simulink model "Fig-6-7-8"  (R2020b)
settings: Solver=VariableStepAuto  StartTime=0.0  StopTime=10.0  RelTol=1e-3
undefined symbols (not defined in the file or in its folder): drv, ms22g, sens, Ts
settings Model: Creator=piera  LastModifiedBy=piera

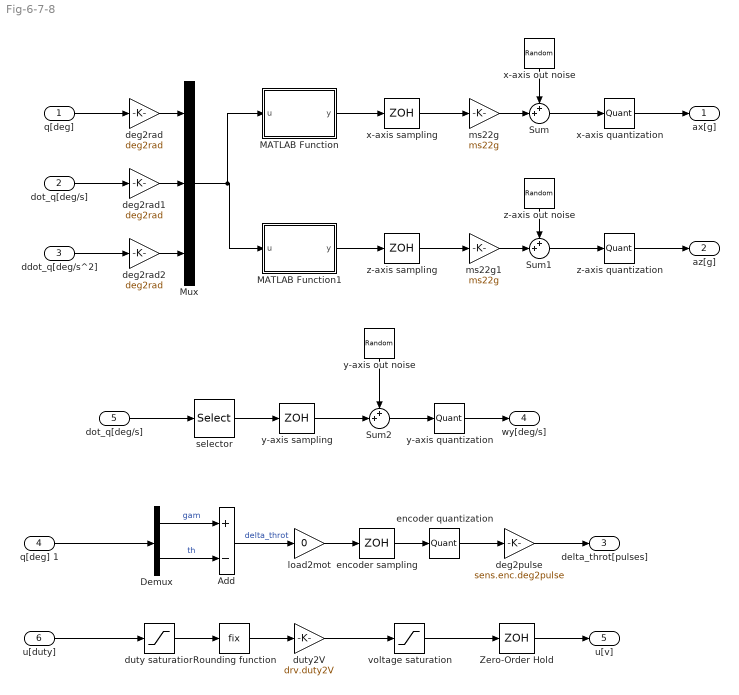
== system Fig-6-7-8 ==
  "q[deg] " : Inport
  dot_q[deg/s] : Inport  Port=2
  ddot_q[deg/s^2] : Inport  Port=3
  q[deg] 1 : Inport  Port=4
  "dot_q[deg/s] " : Inport  Port=5
  u[duty] : Inport  Port=6
  Add : Sum  Inputs=+-
  Demux : Demux  Outputs=2
  MATLAB Function : MATLAB Function  TreatAsAtomicUnit=on
  MATLAB Function1 : MATLAB Function  TreatAsAtomicUnit=on
  Mux : Mux  Inputs=3
  Rounding function : Rounding  Operator=fix
  Sum : Sum  Inputs=++|
  Sum1 : Sum  Inputs=++|
  Sum2 : Sum  Inputs=++|
  Zero-Order Hold : ZeroOrderHold  SampleTime=Ts
  deg2pulse : Gain  Gain=sens.enc.deg2pulse
  deg2rad : Gain  Gain=deg2rad
  deg2rad1 : Gain  Gain=deg2rad
  deg2rad2 : Gain  Gain=deg2rad
  duty saturation : Saturate  UpperLimit=drv.dutymax  LowerLimit=-drv.dutymax
  duty2V : Gain  Gain=drv.duty2V
  encoder quantization : Quantizer  QuantizationInterval=sens.enc.pulse2deg
  encoder sampling : ZeroOrderHold  SampleTime=Ts
  load2mot : Gain  Gain=0
  ms22g : Gain  Gain=ms22g
  ms22g1 : Gain  Gain=ms22g
  selector : Selector  InputPortWidth=2  IndexOptions=Index vector (dialog)  Indices=[2]  OutputSizes=1
  voltage saturation : Saturate  UpperLimit=drv.Vbus  LowerLimit=-drv.Vbus
  x-axis out noise : RandomNumber  Variance=sens.mpu.acc.noisevar  SampleTime=0.1
  x-axis quantization : Quantizer  QuantizationInterval=sens.mpu.acc.LSB2g
  x-axis sampling : ZeroOrderHold  SampleTime=-1
  y-axis out noise : RandomNumber  Variance=sens.mpu.gyro.noisevar  SampleTime=0.1
  y-axis quantization : Quantizer  QuantizationInterval=sens.mpu.gyro.LSB2g
  y-axis sampling : ZeroOrderHold  SampleTime=-1
  z-axis out noise : RandomNumber  Variance=sens.mpu.acc.noisevar  SampleTime=0.1
  z-axis quantization : Quantizer  QuantizationInterval=sens.mpu.acc.LSB2g
  z-axis sampling : ZeroOrderHold  SampleTime=-1
  ax[g] : Outport
  az[g] : Outport  Port=2
  delta_throt[pulses] : Outport  Port=3
  wy[deg/s] : Outport  Port=4
  u[v] : Outport  Port=5
  wires:
  deg2rad1/1 -> Mux/2
  deg2rad/1 -> Mux/1
  deg2rad2/1 -> Mux/3
  "q[deg] "/1 -> deg2rad/1
  dot_q[deg/s]/1 -> deg2rad1/1
  ddot_q[deg/s^2]/1 -> deg2rad2/1
  Mux/1 -> MATLAB Function/1(u), MATLAB Function1/1(u)
  MATLAB Function1/1(y) -> z-axis sampling/1
  MATLAB Function/1(y) -> x-axis sampling/1
  z-axis sampling/1 -> ms22g1/1
  x-axis sampling/1 -> ms22g/1
  ms22g/1 -> Sum/2
  x-axis out noise/1 -> Sum/1
  Sum/1 -> x-axis quantization/1
  x-axis quantization/1 -> ax[g]/1
  z-axis quantization/1 -> az[g]/1
  z-axis out noise/1 -> Sum1/1
  ms22g1/1 -> Sum1/2
  Sum1/1 -> z-axis quantization/1
  deg2pulse/1 -> delta_throt[pulses]/1
  encoder quantization/1 -> deg2pulse/1
  encoder sampling/1 -> encoder quantization/1
  load2mot/1 -> encoder sampling/1
  Add/1 -> load2mot/1  "delta_throt"
  q[deg] 1/1 -> Demux/1
  Demux/1 -> Add/1  "gam"
  Demux/2 -> Add/2  "th"
  y-axis quantization/1 -> wy[deg/s]/1
  Sum2/1 -> y-axis quantization/1
  y-axis out noise/1 -> Sum2/1
  y-axis sampling/1 -> Sum2/2
  selector/1 -> y-axis sampling/1
  "dot_q[deg/s] "/1 -> selector/1
  Zero-Order Hold/1 -> u[v]/1
  voltage saturation/1 -> Zero-Order Hold/1
  duty2V/1 -> voltage saturation/1
  Rounding function/1 -> duty2V/1
  duty saturation/1 -> Rounding function/1
  u[duty]/1 -> duty saturation/1

== matlab function Fig-6-7-8/MATLAB Function ==
  data: u input; y output
function y = fcn(u)

y = u;

== matlab function Fig-6-7-8/MATLAB Function1 ==
  data: u input; y output
function y = fcn(u)

y = u;
